simulink model "Ex9_12model"  (R2013a)
settings: Solver=ode15s  StartTime=0.0  StopTime=800  FixedStep=.001  RelTol=1e-3
settings Model: Creator=John  LastModifiedBy=John

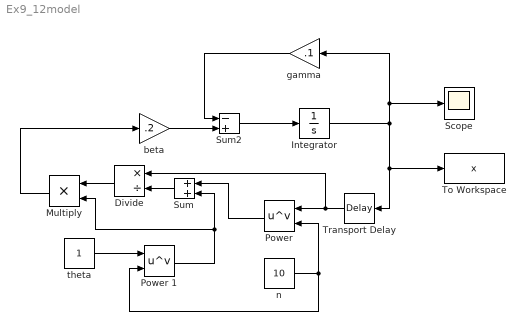
== system Ex9_12model ==
  Divide : Product  Inputs=*/
  Integrator : Integrator  InitialCondition=0.1
  Multiply : Product
  Power : Math  Operator=pow  SaturateOnIntegerOverflow=on
  Power 1 : Math  Operator=pow  SaturateOnIntegerOverflow=on
  Scope : Scope
  Sum : Sum  Inputs=|++
  Sum2 : Sum  Inputs=-+
  To Workspace : ToWorkspace  VariableName=x  SampleTime=-1
  Transport Delay : TransportDelay  DelayTime=20
  beta : Gain  Gain=.2
  gamma : Gain  Gain=.1
  n : Constant  Value=10
  theta : Constant
  wires:
  n/1 -> Power 1/2, Power/2
  Transport Delay/1 -> Divide/1, Power/1
  theta/1 -> Power 1/1
  Power 1/1 -> Multiply/2, Sum/2
  Sum/1 -> Divide/2
  Divide/1 -> Multiply/1
  Multiply/1 -> beta/1
  gamma/1 -> Sum2/1
  beta/1 -> Sum2/2
  Sum2/1 -> Integrator/1
  Integrator/1 -> Transport Delay/1, To Workspace/1, Scope/1, gamma/1
  Power/1 -> Sum/1
